simulink model "rt_test_simple"  (R2019b)
settings: Solver=ode5  StartTime=0.0  StopTime=20  RelTol=1e-3
undefined symbols (not defined in the file): Standard_Devices, UDP_Protocol
libraries: sldrtlib x2, fod x1
settings Model: SimulationMode=external  Creator=Aleksei  LastModifiedBy=Aleksei
settings DataIOCC: ReturnWorkspaceOutputs=off
settings DebuggingCC: ArithmeticOperatorsInVariantConditions=warning
settings SFSimCC: CustomCodeUndefinedFunction=UseInterfaceOnly
settings RTWCC: Description=Simulink Desktop Real-Time  SystemTargetFile=sldrt.tlc  TemplateMakefile=sldrt.tmf  RTWCompilerOptimization=on
settings CodeAppCC: MaxIdLength=95
settings SimulinkDesktopRealTimeCC: TargetPreCompLibLocation=C:\Program Files\MATLAB\R2019b\toolbox\sldrt\lib\win64  PreserveStateflowLocalDataDimensions=off

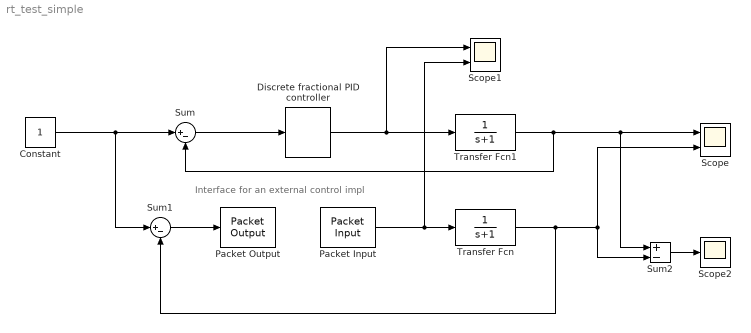
== system rt_test_simple ==
  note: Interface for an external control impl
  Constant : Constant
  Discrete fractional PID controller : fod/Discrete fractional PID controller  Kp=-0.01  Ki=0.25  lambda=0.8  Kd=0.05  mu=0.6  freqRange=[0.001; 1000]  N=5  useRef=off  dscrMethod=Matched  wc=0  ts=0.01
      settings: SourceProductName=FOMCON Toolbox
  Packet Input : sldrtlib/Packet Input  SampleTime=0.01  MaxMissedTicks=10  ShowMissedTicks=off  YieldWhenWaiting=off  DrvName=Standard_Devices/UDP_Protocol  DrvAddress=5101  DrvOptions=[0 5111 49 50 55 46 48 46 48 46 49 0 0 0 0 0 0 0 0 0 0 0 0 0 0 0 0 0 0 0 0 0 0 0 0 0 0 0 0 0 0 0 0 0 0 0 0 0 0 0 0 0 0 0 0 0 0 0 0 0 0 0 0 0 0 0 0 0 0 0 0 0 0 0 0 0 0 0 0 0 0 0 0 0 0 0 0 0 0 0 0 0 0 0 0 0 0 0 0 0 0 0 0 0 0 0 0 0 0 0 0 0 0 0 0 0 0 0 0 0 0 0 0 0 0 0 0 0 0 0 0 0 0 0 0 0 0 0 0 0 0 0 0 0 0 0 0 0 0 0 0 0 0 0 0 0 0 0 0 0 0 0 0 0 0 0 0 0 0 0 0 0 0 0 0 0 0 0 0 0 0 0 0 0 0 0 0 0 0 0 0 0 0 0 0 0 0 0 0 0 0 0 0 0 0 0 0 0 0 0 0 0 0 0 0 0 0 0 0 0 0 0 0 0 0 0 0 0 0 0 0 0 0 0 0 0 0 0 0 0 0 0 0 0 0 0 0 0 0 0 0 0 0 0 0 0]  PacketSize=8  DataTypes='1*double'  ShowReady=off  ShowError=off  PacketID=1  ByteOrder=1  ShowTimestamp=off
      settings: AttributesFormatString=UDP Protocol [5101]  SourceProductName=Simulink Desktop Real-Time
  Packet Output : sldrtlib/Packet Output  SampleTime=0.01  MaxMissedTicks=10  ShowMissedTicks=off  YieldWhenWaiting=off  DrvName=Standard_Devices/UDP_Protocol  DrvAddress=5100  DrvOptions=[0 5110 49 50 55 46 48 46 48 46 49 0 0 0 0 0 0 0 0 0 0 0 0 0 0 0 0 0 0 0 0 0 0 0 0 0 0 0 0 0 0 0 0 0 0 0 0 0 0 0 0 0 0 0 0 0 0 0 0 0 0 0 0 0 0 0 0 0 0 0 0 0 0 0 0 0 0 0 0 0 0 0 0 0 0 0 0 0 0 0 0 0 0 0 0 0 0 0 0 0 0 0 0 0 0 0 0 0 0 0 0 0 0 0 0 0 0 0 0 0 0 0 0 0 0 0 0 0 0 0 0 0 0 0 0 0 0 0 0 0 0 0 0 0 0 0 0 0 0 0 0 0 0 0 0 0 0 0 0 0 0 0 0 0 0 0 0 0 0 0 0 0 0 0 0 0 0 0 0 0 0 0 0 0 0 0 0 0 0 0 0 0 0 0 0 0 0 0 0 0 0 0 0 0 0 0 0 0 0 0 0 0 0 0 0 0 0 0 0 0 0 0 0 0 0 0 0 0 0 0 0 0 0 0 0 0 0 0 0 0 0 0 0 0 0 0 0 0 0 0 0 0 0 0 0 0]  PacketSize=8  DataTypes='1*double'  ShowReady=off  ShowError=off  PacketID=1  ByteOrder=1  InitialValue=[]  FinalValue=[]
      settings: AttributesFormatString=UDP Protocol [5100]  SourceProductName=Simulink Desktop Real-Time
  Scope : Scope  NumInputPorts=2
  Scope1 : Scope  NumInputPorts=2
  Scope2 : Scope
  Sum : Sum  Inputs=|+-
  Sum1 : Sum  Inputs=|+-
  Sum2 : Sum  Inputs=+-
  Transfer Fcn : TransferFcn  Denominator=[1 1]
  Transfer Fcn1 : TransferFcn  Denominator=[1 1]
  wires:
  Transfer Fcn/1 -> Sum1/2, Scope/2, Sum2/2
  Transfer Fcn1/1 -> Sum/2, Sum2/1, Scope/1
  Constant/1 -> Sum1/1, Sum/1
  Sum1/1 -> Packet Output/1
  Packet Input/1 -> Scope1/2, Transfer Fcn/1
  Discrete fractional PID controller/1 -> Scope1/1, Transfer Fcn1/1
  Sum/1 -> Discrete fractional PID controller/1
  Sum2/1 -> Scope2/1
